simulink model "power_windgen_v2"  (R2021a)
settings: Solver=ode23tb  StartTime=0.0  StopTime=5  RelTol=1e-4  EnableMultiTasking=on
PostLoadFcn:
  | find_system (gcs, 'LookUnderMasks', 'all', 'FollowLinks', 'on');
InitFcn:
  | [xInitial,psbwindgen_char] = init_power_windgen;
undefined symbols (not defined in the file): DiscIntNeverNeededParam, psbwindgen_char
libraries: spsIdealSwitchLib x24, spsThreePhaseParallelRLCLoadLib x11, spsThreePhaseVIMeasurementLib x4, spsPower3phInstantaneousLib x4, spsThreePhaseBreakerLib x1, spsAsynchronousMachinepuUnitsLib x1, spsPLL3phLib x1, spsExcitationSystemLib x1, spsSynchronousMachinepuStandardLib x1, spspowerguiLib x1
Description:
  | The Model initialization function Callback automatically
  | 
  | loads the initial states vector xInitial and the wind turbine
  | 
  | characteristics. The initial conditions are stored in the
  | 
  | power_windgen.mat file.
settings Model: ExtModeAutoUpdateStatusClock=off  Creator=The MathWorks, Inc.  LastModifiedBy=enes_
settings SolverCC: AlgebraicLoopSolver=TrustRegion
settings DataIOCC: LoadInitialState=on  SaveFormat=StructureWithTime  SaveOutput=off  SaveTime=off  ReturnWorkspaceOutputs=off  SignalLoggingName=sigsOut
settings OptimizationCC: BlockReduction=off  BooleanDataType=off  ExpressionDepthLimit=2147483647  InitFltsAndDblsToZero=on  EfficientMapNaN2IntZero=off  LifeSpan=inf
settings DebuggingCC: UnderspecifiedInitializationDetection=Classic  MergeDetectMultiDrivingBlocksExec=none  CheckExecutionContextPreStartOutputMsg=on  SignalResolutionControl=TryResolveAllWithWarning  MultiTaskDSMMsg=warning  MultiTaskCondExecSysMsg=none  FcnCallInpInsideContextMsg=warning  AllowSymbolicDim=off  StateNameClashWarn=warning  SFUnexpectedBacktrackingDiag=warning  SFNoUnconditionalDefaultTransitionDiag=warning  SFExecutionAtInitializationDiag=none  SFMachineParentedDataDiag=warning  ArithmeticOperatorsInVariantConditions=warning
settings HardwareCC: ProdBitPerPointer=32  ProdBitPerSizeT=32  ProdBitPerPtrDiffT=32  ProdLargestAtomicFloat=None  ProdIntDivRoundTo=Undefined  ProdEndianess=Unspecified  ProdWordSize=32  ProdHWDeviceType=Specified  TargetUnknown=on
settings ModelReferenceCC: PropagateSignalLabelsOutOfModel=off
settings SFSimCC: SimUseLocalCustomCode=off  CustomCodeUndefinedFunction=UseInterfaceOnly
settings RTWCC: RTWUseLocalCustomCode=off
settings CodeAppCC: StateflowObjectComments=on
settings GRTTargetCC: TargetLangStandard=C89/C90 (ANSI)  CombineOutputUpdateFcns=off  GRTInterface=on
settings ConfigComp: CovMetricSettings=dw  CovSaveCumulativeToWorkspaceVar=on  CovSaveSingleToWorkspaceVar=on  CovExternalEMLEnable=off  CovSFcnEnable=off
settings SimscapeCC: SimscapeNormalizeSystem=off

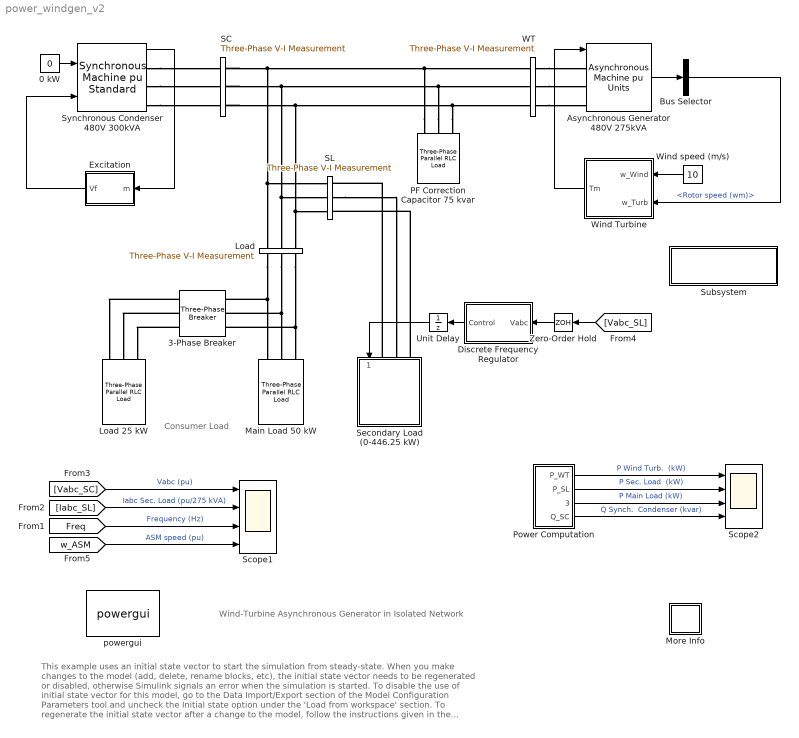
== system power_windgen_v2 ==
  note: This example uses an initial state vector to start the simulation from steady-state. When you make changes to the model (add, delete, rename blocks, etc),
      | the initial state vector needs to be regenerated or disabled, otherwise Simulink signals an error when the simulation is started.
      | To disable the use of initial state vector for this model, go to the Data Import/Export section of the Model Configuration Parameters tool and uncheck the
      | Initial state option under the 'Load from workspace' section.
      | To regenerate the initial state vector after a change to the model, follow the instructions given in the initialization file for this model.
      | Type open('init_power_windgen') at the matlab prompt to view this file.
  note: Wind-Turbine Asynchronous Generator in Isolated Network
  note: Consumer Load
  0 kW : Constant  Value=0
  3-Phase Breaker : spsThreePhaseBreakerLib/Three-Phase Breaker  InitialState=open  SwitchA=on  SwitchB=on  SwitchC=on  SwitchTimes=[0.2]  External=off  BreakerResistance=0.001  SnubberResistance=1e6  SnubberCapacitance=inf  Measurements=None
      settings: AttributesFormatString=\n
  Asynchronous Generator 480V 275kVA : spsAsynchronousMachinepuUnitsLib/Asynchronous Machine pu Units  RotorType=Squirrel-cage  PresetModel=No  MechanicalLoad=Torque Tm  ShowDetailedParameters=on  ReferenceFrame=Rotor  Units=pu  MeasurementBus=off  NominalParameters=[ 275e3, 480, 60 ]  VoltageRatio=1  Stator=[ 0.016,0.06]  Rotor=[ 0.015,0.06]  Cage1=[0.01909 0.0397]  Cage2=[0.01909 0.0397]  Lm=3.5  Mechanical=[ 2,0,2 ]  PolePairs=2  InitialConditions=[-8.89496e-048 0 0.280896 0.280896 0.280896 -89.7425 150.258 30.2575]  SimulateSaturation=off  Saturation=[ 0 0 ; 0 0 ]  LoadFlowParameters=0  TsPowergui=0  TsBlock=-1  IterativeModel=Trapezoidal non iterative  IterativeDiscreteModel=Trapezoidal non iterative  Pmec=0
      settings: AttributesFormatString=\n  SourceProductBaseCode=PS
  Bus Selector : BusSelector  OutputSignals=Mechanical.Rotor speed (wm)
  Discrete Frequency Regulator : Subsystem  mask(Discrete Frequency Regulator){Freq_ref=60, gains_regulator=[255 30], Vpp_nom=480, Ts=200e-6}
      mask prompts: Freq_ref "Reference frequency (Hz):"; gains_regulator "Regulator gains  [Kp Kd]:"; Vpp_nom "Phase to phase voltage (Vrms):"; Ts "Sample time (s):"
      mask help:
      | Input : phase to ground voltages
      |
      | Output : 24 logical signals for the control of the dump load
      mask init:
      | Vbase=Vpp_nom/sqrt(3);
      | Kp=gains_regulator(1);
      | Kd=gains_regulator(2);
  Excitation : Subsystem
  Load : spsThreePhaseVIMeasurementLib/Three-Phase V-I Measurement  VoltageMeasurement=phase-to-ground  SetLabelV=on  LabelV=Vabc_Load  Vpu=on  VpuLL=off  CurrentMeasurement=yes  SetLabelI=on  LabelI=Iabc_Load  Ipu=on  Pbase=275e3  Vbase=480  OutputType=Magnitude  PhasorSimulation=off  PSBequivalent=0
  Load 25 kW : spsThreePhaseParallelRLCLoadLib/Three-Phase Parallel RLC Load  LConnTagsString=A|B|C  Configuration=Y (grounded)  NominalVoltage=480  Vabc=[1e3 1e3 1e3]  Vabcp=[1e3 1e3 1e3]  NominalFrequency=60  UnbalancedPower=off  ActivePower=25e3  InductivePower=0  CapacitivePower=0  Pabc=[10e3 9e3 11e3]  QLabc=[100 90 110]  QCabc=[100 90 110]  Pabcp=[10e3 9e3 11e3]  QLabcp=[100 90 110]  QCabcp=[100 90 110]  Measurements=None  LoadType=constant Z
  Main Load 50 kW : spsThreePhaseParallelRLCLoadLib/Three-Phase Parallel RLC Load  LConnTagsString=A|B|C  Configuration=Y (grounded)  NominalVoltage=480  Vabc=[1e3 1e3 1e3]  Vabcp=[1e3 1e3 1e3]  NominalFrequency=60  UnbalancedPower=off  ActivePower=50e3  InductivePower=0  CapacitivePower=0  Pabc=[10e3 9e3 11e3]  QLabc=[100 90 110]  QCabc=[100 90 110]  Pabcp=[10e3 9e3 11e3]  QLabcp=[100 90 110]  QCabcp=[100 90 110]  Measurements=None  LoadType=constant Z
  More Info : Subsystem
      settings: OpenFcn=showdemo(bdroot(gcb))
      mask Display: disp('?')
  PF Correction Capacitor 75 kvar : spsThreePhaseParallelRLCLoadLib/Three-Phase Parallel RLC Load  LConnTagsString=A|B|C  Configuration=Delta  NominalVoltage=480  Vabc=[1e3 1e3 1e3]  Vabcp=[1e3 1e3 1e3]  NominalFrequency=60  UnbalancedPower=off  ActivePower=0  InductivePower=0  CapacitivePower=75e3  Pabc=[10e3 9e3 11e3]  QLabc=[100 90 110]  QCabc=[100 90 110]  Pabcp=[10e3 9e3 11e3]  QLabcp=[100 90 110]  QCabcp=[100 90 110]  Measurements=None  LoadType=constant Z
  Power Computation : Subsystem
  SC : spsThreePhaseVIMeasurementLib/Three-Phase V-I Measurement  VoltageMeasurement=phase-to-ground  SetLabelV=on  LabelV=Vabc_SC  Vpu=on  VpuLL=off  CurrentMeasurement=yes  SetLabelI=on  LabelI=Iabc_SC  Ipu=on  Pbase=300e3  Vbase=480  OutputType=Magnitude  PhasorSimulation=off  PSBequivalent=0
  SL : spsThreePhaseVIMeasurementLib/Three-Phase V-I Measurement  VoltageMeasurement=phase-to-ground  SetLabelV=on  LabelV=Vabc_SL  Vpu=on  VpuLL=off  CurrentMeasurement=yes  SetLabelI=on  LabelI=Iabc_SL  Ipu=on  Pbase=275e3  Vbase=480  OutputType=Magnitude  PhasorSimulation=off  PSBequivalent=0
  Scope1 : Scope  NumInputPorts=4
  Scope2 : Scope  NumInputPorts=4
  Secondary Load (0-446.25 kW) : Subsystem  mask(8-step Variable Load){Vphase_phase_lissage=480, Freq=60, P_lissage_min=1.75e3, Pin_3phase=50e3}
      mask prompts: Vphase_phase_lissage "Nominal L-L voltage (Vrms):"; Freq "Nominal frequency (Hz):"; P_lissage_min "Power per step Pstep (W):"; Pin_3phase "Initial power  (W) :"
      mask help:
      | This block implements a variable, three-phase resistive load. The load variation uses an eight-bit binary progression so that the load power can be varied by steps from 0 to 255*Pstep.
      |
      | The eight three-phase resistors are connected in series with ideal switches simulating forced-commutated power electronic switches.
      |
      | The Pulses input is a vector containing the eight bits (0/1) controlling the eight three-phase switches. First value is the less significant bit.
      mask init:
      | Ron_switch=1e-6;
      | Rs_snubber=inf;
      | Cs_snubber=0;
      | n_niveaux=8;
      | Pmax=((2^n_niveaux)-1)*P_lissage_min;
      | Pin_normalise=min([(Pin_3phase/Pmax)*((2^n_niveaux)-1) ((2^n_niveaux)-1)]);
      | discret1=pow2(0:-1:-(n_niveaux-1))*Pin_normalise;
      | discret2=floor(discret1);
      | Status=rem(discret2,2);
  Subsystem : Subsystem
      settings: OpenFcn=open('psbwindgen_turb.fig')
      mask Display: disp('Double click to display\nTurbine characteristics')
  Synchronous Condenser 480V 300kVA : spsSynchronousMachinepuStandardLib/Synchronous Machine pu Standard  PresetModel=No  MechanicalLoad=Mechanical power Pm  ShowDetailedParameters=on  RotorType=Salient-pole  Units=per unit standard parameters  MeasurementBus=off  NominalParameters=[ 300e3 480 60 ]  Reactances1=[ 3.23, 0.21, 0.15, 2.79, 1.03, 0.37, 0.09 ]  Reactances2=[2.24 0.17 0.12 1.02 0.13 0.08]  dAxisTimeConstants=Open-circuit  qAxisTimeConstants=Open-circuit  TimeConstants1="[ 4.4849  0.0681  0.1  ]"  TimeConstants2=[ 1.7, 0.008, 0.213, 0.004 ]  TimeConstants3="[  1.7 0.008 0.051266  ]"  TimeConstants4=[ 8.0, 0.03, 0.3371, 0.0295 ]  TimeConstants5="[ 0.08  0.019  0.004 ]"  TimeConstants6=[ 1.3201, 0.023, 1.0, 0.07 ]  TimeConstants7="[  0.08  0.019 0.051266  ]"  TimeConstants8=[ 1.3201, 0.0231, 0.3371, 0.0295 ]  StatorResistance=0.017  Mechanical=[ 1, 0, 2 ]  PolePairs=2  InitialConditions=[0 -89.2146 0.827 0.827 0.827 -86.4 153.6 33.6 2.71455]  SetSaturation=off  Saturation=[0.6404,0.7127,0.8441,0.9214,0.9956,1.082,1.19,1.316,1.457;0.7,0.7698,0.8872,0.9466,0.9969,1.046,1.1,1.151,1.201]  LoadFlowParameters=[2 0 0 0 0]  TsPowergui=0  TsBlock=-1  IterativeModel=Trapezoidal non iterative  IterativeDiscreteModel=Trapezoidal non iterative  BusType=PV  Pref=0  Qref=0  Qmin=-inf  Qmax=inf  PLF=0  QLF=0
      settings: SourceProductBaseCode=PS
  Unit Delay : UnitDelay  SampleTime=200e-6  HasFrameUpgradeWarning=on
  WT : spsThreePhaseVIMeasurementLib/Three-Phase V-I Measurement  VoltageMeasurement=phase-to-ground  SetLabelV=on  LabelV=Vabc_WT  Vpu=on  VpuLL=off  CurrentMeasurement=yes  SetLabelI=on  LabelI=Iabc_WT  Ipu=on  Pbase=275e3  Vbase=480  OutputType=Magnitude  PhasorSimulation=off  PSBequivalent=0
  Wind Turbine : Subsystem
  Wind speed (m/s) : Constant  Value=10
  Zero-Order Hold : ZeroOrderHold  SampleTime=200e-6
  powergui : spspowerguiLib/powergui  SimulationMode=Continuous  SampleTime=0  frequency=60  Iterations=50  frequencyindice=60  Pbase=100e6  ErrMax=1e-4  UnitsV=kV  UnitsW=MW  buscounter=0  FunctionMessages=off  echomessages=off  EnableUseOfTLC=off  CurrentSourceSwitches=on  DisableSnubberDevices=on  DisableRonSwitches=off  DisableVfSwitches=off  DisplayEquations=off  AutomaticDiscreteSolvers=off  SolverType=Tustin  Interpol=off  ExternalGateDelay=off  methode=off  Ts=0  x0status=blocks  SPID=off  SwTol=0  HookPort=off  NonlinearTolerance=1e-4  nMaxIteration=100  ContinueOnMaxIteration=off  RestoreLinks=warning  ResistiveCurrentMeasurement=off  Frange=[0:2:500]  Ylog=off  Xlog=on  ShowGrid=off  save=off  variable=ZData  structure=0  ZoomFFT=on  StartTime=0.0  cycles=1  DisplayStyle=1  fundamental=60  FreqAxis=off  MaxFrequency=1000  frequencyindicesteady=1  RmsSteady=1  display=off
  wires:
  [Freq] -> Scope1/3  "Frequency (Hz)"
  [Vabc_SC] -> Scope1/1  "Vabc (pu)"
  [Iabc_SL] -> Scope1/2  "Iabc Sec. Load (pu/275 kVA)"
  Wind speed (m/s)/1 -> Wind Turbine/1(w_Wind)
  [Vabc_SL] -> Zero-Order Hold/1
  Power Computation/1(P_WT) -> Scope2/1  "P Wind Turb.  (kW)"
  Power Computation/2(P_SL) -> Scope2/2  "P Sec. Load  (kW)"
  Power Computation/3(P_Load) -> Scope2/3  "P Main Load (kW)"
  Power Computation/4(Q_SC) -> Scope2/4  "Q Synch.  Condenser (kvar)"
  Discrete Frequency Regulator/1(Control) -> Unit Delay/1
  [w_ASM] -> Scope1/4  "ASM speed (pu)"
  0 kW/1 -> Synchronous Condenser 480V 300kVA/1
  Synchronous Condenser 480V 300kVA/1 -> Excitation/1(m)
  Excitation/1(Vf) -> Synchronous Condenser 480V 300kVA/2
  Asynchronous Generator 480V 275kVA/1 -> Bus Selector/1
  Wind Turbine/1(Tm) -> Asynchronous Generator 480V 275kVA/1
  Bus Selector/1 -> Wind Turbine/2(w_Turb)  "<Rotor speed (wm)>"
  Unit Delay/1 -> Secondary Load (0-446.25 kW)/1(Control)
  Zero-Order Hold/1 -> Discrete Frequency Regulator/1(Vabc)
  connections:
  Load/RConn3 -- Main Load 50 kW/LConn3 -- 3-Phase Breaker/LConn3
  Load/RConn1 -- Main Load 50 kW/LConn1 -- 3-Phase Breaker/LConn1
  Load/RConn2 -- Main Load 50 kW/LConn2 -- 3-Phase Breaker/LConn2
  WT/RConn1 -- Asynchronous Generator 480V 275kVA/LConn1
  WT/RConn2 -- Asynchronous Generator 480V 275kVA/LConn2
  WT/RConn3 -- Asynchronous Generator 480V 275kVA/LConn3
  Synchronous Condenser 480V 300kVA/RConn1 -- SC/LConn1
  Synchronous Condenser 480V 300kVA/RConn2 -- SC/LConn2
  Synchronous Condenser 480V 300kVA/RConn3 -- SC/LConn3
  PF Correction Capacitor 75 kvar/LConn1 -- WT/LConn1 -- SC/RConn1 -- Load/LConn1 -- SL/LConn1
  PF Correction Capacitor 75 kvar/LConn2 -- WT/LConn2 -- SC/RConn2 -- Load/LConn2 -- SL/LConn2
  PF Correction Capacitor 75 kvar/LConn3 -- WT/LConn3 -- SC/RConn3 -- Load/LConn3 -- SL/LConn3
  3-Phase Breaker/RConn1 -- Load 25 kW/LConn1
  3-Phase Breaker/RConn2 -- Load 25 kW/LConn2
  3-Phase Breaker/RConn3 -- Load 25 kW/LConn3
  Secondary Load (0-446.25 kW)/LConn1 -- SL/RConn1
  SL/RConn2 -- Secondary Load (0-446.25 kW)/LConn2
  Secondary Load (0-446.25 kW)/LConn3 -- SL/RConn3

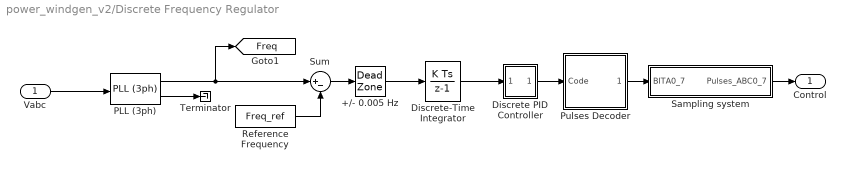
== system power_windgen_v2/Discrete Frequency Regulator ==
  Vabc : Inport
  +/- 0.005 Hz : DeadZone  LowerValue=-0.005  UpperValue=0.005  SaturateOnIntegerOverflow=on
  Discrete PID Controller : Subsystem  DialogController=POWERSYS.PowerSysDialog  mask(Discrete PID Controller){Kp=Kp, Ki=0, Kd=Kd, TcD=0.5e-3, Par_Limits=[255 0], Init=0, Ts=Ts}
      mask prompts: Kp "Proportional gain (Kp):"; Ki "Integral gain (Ki):"; Kd "Derivative gain (Kd):"; TcD "Time constant for derivative (s):"; Par_Limits "Output limits: [ Upper   Lower ]"; Init "Output initial value:"; Ts "Sample time:"
      mask help: This block implements a discrete PID controller.
      mask init:
      | UpperLimit=Par_Limits(1);
      | LowerLimit=Par_Limits(2);
      | power_initmask();
      mask Help: This block is part of a subset of blocks in the Extras library that does not have documentation associated with it, other than the block mask description.
      mask Display: disp('PID');
  Discrete-Time Integrator : DiscreteIntegrator  SampleTime=Ts  LimitOutput=on  UpperSaturationLimit=1  LowerSaturationLimit=0  ICPrevOutput=DiscIntNeverNeededParam  ICPrevScaledInput=DiscIntNeverNeededParam
  PLL (3ph) : spsPLL3phLib/PLL (3ph)  Fmin=45  Par_Init=[0 Freq_ref]  ParK=[60 1400]  TcD=2e-4  MaxRateChangeFreq=12  FilterCutOffFreq=25  Ts=Ts  AGC=on
  Pulses Decoder : Subsystem  mask(Pulses Decoder){n=8}
      mask prompts: n "Number of bits to decode:"
      mask help:
      | Decode the scalar input 'Code' into a vector output 'Pulses' based on  the specified number of bits to decode.
      | (Element 1 of vector output = least significant bit)
  Reference Frequency : Constant  Value=Freq_ref
  Sampling system : Subsystem
  Sum : Sum  Inputs=|+-  InputSameDT=on  SaturateOnIntegerOverflow=on  OutDataTypeStr=Inherit: Same as first input
  Terminator : Terminator
  Control : Outport  VectorParamsAs1DForOutWhenUnconnected=off
  tag scope: Freq=global
  wires:
  Vabc/1 -> PLL (3ph)/1
  PLL (3ph)/2 -> Terminator/1
  Sampling system/1(Pulses_ABC0_7) -> Control/1
  Discrete-Time Integrator/1 -> Discrete PID Controller/1(Error)
  Reference Frequency/1 -> Sum/2
  Discrete PID Controller/1(Out) -> Pulses Decoder/1(Code)
  Sum/1 -> +/- 0.005 Hz/1
  Pulses Decoder/1(Pulses) -> Sampling system/1(BITA0_7)
  +/- 0.005 Hz/1 -> Discrete-Time Integrator/1
  PLL (3ph)/1 -> Sum/1, [Freq]

== system power_windgen_v2/Excitation ==
  m : Inport
  Bus Selector1 : BusSelector  OutputSignals="dq0 components.Stator voltage  vd (pu),dq0 components.Stator voltage  vq (pu)"
  Constant3 : Constant
  Excitation System : spsExcitationSystemLib/Excitation System  tr=20e-3  reg=[ 300, 0.001 ]  exc=[ 1, 0 ]  tgr=[ 0, 0 ]  damp=[ 0.001, 0.1 ]  sat=[ 0, 0 ]  lim=[ -11.5, 11.5, 0 ]  v0=[1,2.71455]
      settings: SourceProductBaseCode=PS
  Ground : Ground
  Vf : Outport  VectorParamsAs1DForOutWhenUnconnected=off
  wires:
  Constant3/1 -> Excitation System/1
  Ground/1 -> Excitation System/4
  m/1 -> Bus Selector1/1
  Excitation System/1 -> Vf/1
  Bus Selector1/1 -> Excitation System/2  "<Stator voltage  vd (pu)>"
  Bus Selector1/2 -> Excitation System/3  "<Stator voltage  vq (pu)>"

== system power_windgen_v2/More Info ==

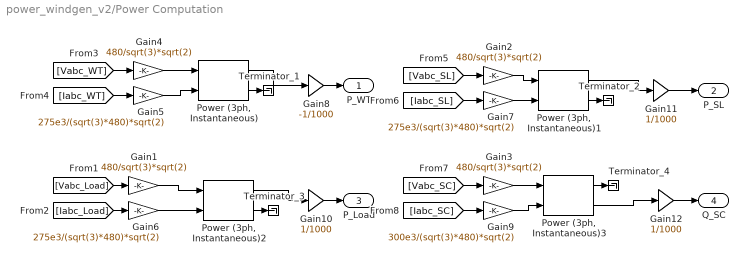
== system power_windgen_v2/Power Computation ==
  Gain{1..4} (4 alike) : Gain  Gain=480/sqrt(3)*sqrt(2)  SaturateOnIntegerOverflow=on  OutDataTypeStr=Inherit: Same as input  ParamDataTypeStr=Inherit: Same as input
  Gain10 : Gain  Gain=1/1000  SaturateOnIntegerOverflow=on  OutDataTypeStr=Inherit: Same as input  ParamDataTypeStr=Inherit: Same as input
  Gain11 : Gain  Gain=1/1000  SaturateOnIntegerOverflow=on  OutDataTypeStr=Inherit: Same as input  ParamDataTypeStr=Inherit: Same as input
  Gain12 : Gain  Gain=1/1000  SaturateOnIntegerOverflow=on  OutDataTypeStr=Inherit: Same as input  ParamDataTypeStr=Inherit: Same as input
  Gain5 : Gain  Gain=275e3/(sqrt(3)*480)*sqrt(2)  SaturateOnIntegerOverflow=on  OutDataTypeStr=Inherit: Same as input  ParamDataTypeStr=Inherit: Same as input
  Gain6 : Gain  Gain=275e3/(sqrt(3)*480)*sqrt(2)  SaturateOnIntegerOverflow=on  OutDataTypeStr=Inherit: Same as input  ParamDataTypeStr=Inherit: Same as input
  Gain7 : Gain  Gain=275e3/(sqrt(3)*480)*sqrt(2)  SaturateOnIntegerOverflow=on  OutDataTypeStr=Inherit: Same as input  ParamDataTypeStr=Inherit: Same as input
  Gain8 : Gain  Gain=-1/1000  SaturateOnIntegerOverflow=on  OutDataTypeStr=Inherit: Same as input  ParamDataTypeStr=Inherit: Same as input
  Gain9 : Gain  Gain=300e3/(sqrt(3)*480)*sqrt(2)  SaturateOnIntegerOverflow=on  OutDataTypeStr=Inherit: Same as input  ParamDataTypeStr=Inherit: Same as input
  Power (3ph, Instantaneous){,1..3} (4 alike) : spsPower3phInstantaneousLib/Power (3ph, Instantaneous)
  Terminator_{1..4} (4 alike) : Terminator
  P_WT : Outport  VectorParamsAs1DForOutWhenUnconnected=off
  P_SL : Outport  Port=2  VectorParamsAs1DForOutWhenUnconnected=off
  P_Load : Outport  Port=3  VectorParamsAs1DForOutWhenUnconnected=off
  Q_SC : Outport  Port=4  VectorParamsAs1DForOutWhenUnconnected=off
  wires:
  "Power (3ph, Instantaneous)1"/1 -> Gain11/1
  [Vabc_WT] -> Gain4/1
  [Iabc_WT] -> Gain5/1
  Gain4/1 -> "Power (3ph, Instantaneous)"/1
  Gain5/1 -> "Power (3ph, Instantaneous)"/2
  [Vabc_Load] -> Gain1/1
  [Iabc_Load] -> Gain6/1
  Gain1/1 -> "Power (3ph, Instantaneous)2"/1
  Gain6/1 -> "Power (3ph, Instantaneous)2"/2
  [Vabc_SL] -> Gain2/1
  [Iabc_SL] -> Gain7/1
  Gain2/1 -> "Power (3ph, Instantaneous)1"/1
  Gain7/1 -> "Power (3ph, Instantaneous)1"/2
  "Power (3ph, Instantaneous)2"/1 -> Gain10/1
  "Power (3ph, Instantaneous)"/1 -> Gain8/1
  Gain8/1 -> P_WT/1
  "Power (3ph, Instantaneous)3"/2 -> Gain12/1
  [Vabc_SC] -> Gain3/1
  [Iabc_SC] -> Gain9/1
  Gain3/1 -> "Power (3ph, Instantaneous)3"/1
  Gain9/1 -> "Power (3ph, Instantaneous)3"/2
  Gain10/1 -> P_Load/1
  Gain11/1 -> P_SL/1
  Gain12/1 -> Q_SC/1
  "Power (3ph, Instantaneous)"/2 -> Terminator_1/1
  "Power (3ph, Instantaneous)1"/2 -> Terminator_2/1
  "Power (3ph, Instantaneous)2"/2 -> Terminator_3/1
  "Power (3ph, Instantaneous)3"/1 -> Terminator_4/1

== system power_windgen_v2/Secondary Load (0-446.25 kW) ==
  Control : Inport
  Demux : Demux  Outputs=8
      settings: DisplayOption=none
  Resistive Loads : Subsystem
  Switches : Subsystem
  A : PMIOPort  Side=Left
  B : PMIOPort  Port=2  Side=Left
  C : PMIOPort  Port=3  Side=Left
  wires:
  Control/1 -> Demux/1
  Demux/8 -> Switches/8(P_ABC7)
  Demux/7 -> Switches/7(P_ABC6)
  Demux/6 -> Switches/6(P_ABC5)
  Demux/5 -> Switches/5(P_ABC4)
  Demux/4 -> Switches/4(P_ABC3)
  Demux/3 -> Switches/3(P_ABC2)
  Demux/2 -> Switches/2(P_ABC1)
  Demux/1 -> Switches/1(P_ABC0)
  connections:
  Switches/RConn1 -- Resistive Loads/LConn1
  Switches/RConn2 -- Resistive Loads/LConn2
  Switches/RConn3 -- Resistive Loads/LConn3
  Switches/RConn4 -- Resistive Loads/LConn4
  Switches/RConn5 -- Resistive Loads/LConn5
  Switches/RConn6 -- Resistive Loads/LConn6
  Switches/RConn7 -- Resistive Loads/LConn7
  Switches/RConn8 -- Resistive Loads/LConn8
  Switches/RConn9 -- Resistive Loads/LConn9
  Switches/RConn10 -- Resistive Loads/LConn10
  Switches/RConn11 -- Resistive Loads/LConn11
  Switches/RConn12 -- Resistive Loads/LConn12
  Switches/RConn13 -- Resistive Loads/LConn13
  Switches/RConn14 -- Resistive Loads/LConn14
  Switches/RConn15 -- Resistive Loads/LConn15
  Switches/RConn16 -- Resistive Loads/LConn16
  Switches/RConn17 -- Resistive Loads/LConn17
  Switches/RConn18 -- Resistive Loads/LConn18
  Switches/RConn19 -- Resistive Loads/LConn19
  Switches/RConn20 -- Resistive Loads/LConn20
  Switches/RConn21 -- Resistive Loads/LConn21
  Switches/RConn22 -- Resistive Loads/LConn22
  Switches/RConn23 -- Resistive Loads/LConn23
  Switches/RConn24 -- Resistive Loads/LConn24
  A/RConn1 -- Switches/LConn1
  B/RConn1 -- Switches/LConn2
  C/RConn1 -- Switches/LConn3

== system power_windgen_v2/Subsystem ==

== system power_windgen_v2/Wind Turbine ==
  w_Wind : Inport
  w_Turb : Inport  Port=2
  1800 rpm : Gain  Gain=1800  SaturateOnIntegerOverflow=on  OutDataTypeStr=Inherit: Same as input  ParamDataTypeStr=Inherit: Same as input
  Constant3 : Constant  Value=1e-6
  Gain : Gain  Gain=-1  SaturateOnIntegerOverflow=on  OutDataTypeStr=Inherit: Same as input  ParamDataTypeStr=Inherit: Same as input
  P(w_Wind,w_Turb) : Lookup_n-D  BreakpointsForDimension1=[0 5 6 7 8 9 10 11 12]  BreakpointsForDimension2=[0 571.55 685.8 800.15 914.4 1028.8 1143.1 1257.4 1371.7 1486 1600.3 1714.6 1828.9 1943.2 2057.5 2171.8 2286.1 2400.5 2514.7 2629.1 2743.3 2857.7 2971.9 3086.3 3200.5 3314.9 3429.2]  Table=psbwindgen_char  InternalRulePriority=Speed  RndMeth=Simplest  InputSameDT=on
      settings: InputPortMap=u0,u1
  Product : Product  Inputs=*/  InputSameDT=on  SaturateOnIntegerOverflow=on  OutDataTypeStr=Inherit: Same as first input
  Switch : Switch  Threshold=1e-6  SaturateOnIntegerOverflow=on  InputSameDT=on
  Tm : Outport  VectorParamsAs1DForOutWhenUnconnected=off
  tag scope: w_ASM=global
  wires:
  w_Turb/1 -> 1800 rpm/1, Switch/1, Switch/2, [w_ASM]
  Constant3/1 -> Switch/3
  w_Wind/1 -> P(w_Wind,w_Turb)/1
  P(w_Wind,w_Turb)/1 -> Product/1
  Switch/1 -> Product/2
  Product/1 -> Gain/1
  Gain/1 -> Tm/1
  1800 rpm/1 -> P(w_Wind,w_Turb)/2

== system power_windgen_v2/Discrete Frequency Regulator/Discrete PID Controller ==
  note: Pierre Giroux, Gilbert Sybille
      | Power System Simulation Laboratory
      | IREQ, Hydro-Quebc
  note: Discrete PID Controller
  Error : Inport  SampleTime=Ts
  "Derivative " : DiscreteTransferFcn  Numerator=[2 -2]  Denominator=[Ts+2*TcD Ts-2*TcD]  SampleTime=Ts
  Discrete-Time Integrator : DiscreteIntegrator  InitialCondition=Init  SampleTime=Ts  LimitOutput=on  UpperSaturationLimit=UpperLimit  LowerSaturationLimit=LowerLimit  ICPrevOutput=DiscIntNeverNeededParam  ICPrevScaledInput=DiscIntNeverNeededParam
  Kp4 : Gain  Gain=Kp  SaturateOnIntegerOverflow=on  SampleTime=Ts  OutDataTypeStr=Inherit: Same as input  ParamDataTypeStr=Inherit: Same as input
  Kp5 : Gain  Gain=Ki  SaturateOnIntegerOverflow=on  SampleTime=Ts  OutDataTypeStr=Inherit: Same as input  ParamDataTypeStr=Inherit: Same as input
  Kp6 : Gain  Gain=Kd  SaturateOnIntegerOverflow=on  SampleTime=Ts  OutDataTypeStr=Inherit: Same as input  ParamDataTypeStr=Inherit: Same as input
  Saturation2 : Saturate  UpperLimit=UpperLimit  LowerLimit=LowerLimit  SampleTime=Ts
  Sum6 : Sum  Inputs=+++  InputSameDT=on  SaturateOnIntegerOverflow=on  SampleTime=Ts  OutDataTypeStr=Inherit: Same as first input
  Zero-Order Hold : ZeroOrderHold  SampleTime=Ts
  Out : Outport  SampleTime=Ts  InitialOutput=0  VectorParamsAs1DForOutWhenUnconnected=off
  wires:
  Saturation2/1 -> Out/1
  Error/1 -> Kp4/1, Kp5/1, Kp6/1
  Sum6/1 -> Saturation2/1
  Kp5/1 -> Discrete-Time Integrator/1
  Kp6/1 -> "Derivative "/1
  Kp4/1 -> Zero-Order Hold/1
  Discrete-Time Integrator/1 -> Sum6/2
  "Derivative "/1 -> Sum6/3
  Zero-Order Hold/1 -> Sum6/1

== system power_windgen_v2/Discrete Frequency Regulator/Pulses Decoder ==
  Code : Inport
  Constant : Constant  Value=pow2(0:-1:-(n-1))
  Constant6 : Constant  Value=2
  Math Function : Math  Operator=rem  SignedPower=on  SaturateOnIntegerOverflow=on
  Product : Product  InputSameDT=on  SaturateOnIntegerOverflow=on  OutDataTypeStr=Inherit: Same as first input
  Rounding Function : Rounding
  Pulses : Outport  VectorParamsAs1DForOutWhenUnconnected=off
  wires:
  Math Function/1 -> Pulses/1
  Rounding Function/1 -> Math Function/1
  Constant6/1 -> Math Function/2
  Product/1 -> Rounding Function/1
  Code/1 -> Product/1
  Constant/1 -> Product/2

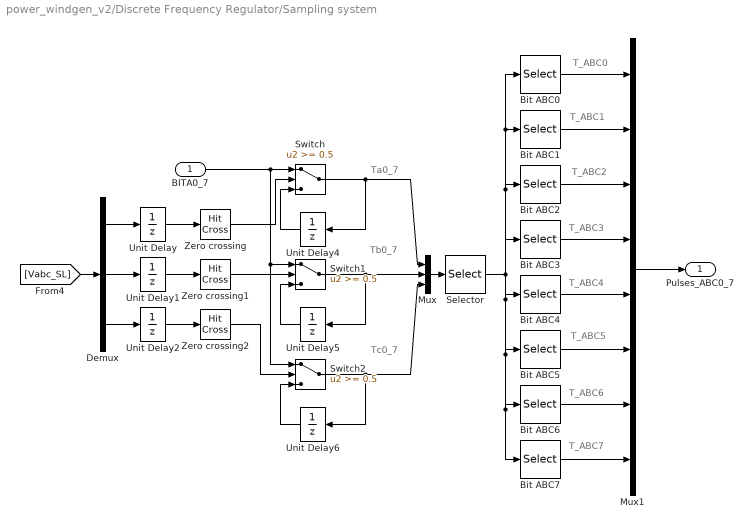
== system power_windgen_v2/Discrete Frequency Regulator/Sampling system ==
  note: T_ABC7
  note: T_ABC6
  note: T_ABC5
  note: T_ABC4
  note: T_ABC3
  note: T_ABC2
  note: T_ABC1
  note: T_ABC0
  note: Tc0_7
  note: Tb0_7
  note: Ta0_7
  BITA0_7 : Inport
  " Bit ABC4" : Selector  InputPortWidth=24  IndexOptions=Index vector (dialog)  Indices=[13 14 15]  OutputSizes=1
  Bit ABC0 : Selector  InputPortWidth=24  IndexOptions=Index vector (dialog)  Indices=[1 2 3]  OutputSizes=1
  Bit ABC1 : Selector  InputPortWidth=24  IndexOptions=Index vector (dialog)  Indices=[4 5 6]  OutputSizes=1
  Bit ABC2 : Selector  InputPortWidth=24  IndexOptions=Index vector (dialog)  Indices=[7 8 9]  OutputSizes=1
  Bit ABC3 : Selector  InputPortWidth=24  IndexOptions=Index vector (dialog)  Indices=[10 11 12]  OutputSizes=1
  Bit ABC5 : Selector  InputPortWidth=24  IndexOptions=Index vector (dialog)  Indices=[16 17 18]  OutputSizes=1
  Bit ABC6 : Selector  InputPortWidth=24  IndexOptions=Index vector (dialog)  Indices=[19 20 21]  OutputSizes=1
  Bit ABC7 : Selector  InputPortWidth=24  IndexOptions=Index vector (dialog)  Indices=[22 23 24]  OutputSizes=1
  Demux : Demux  Outputs=3
      settings: DisplayOption=none
  Mux : Mux  Inputs=3
  Mux1 : Mux  Inputs=8
  Selector : Selector  InputPortWidth=24  IndexOptions=Index vector (dialog)  Indices=[1 9 17 2 10 18 3 11 19 4 12 20 5 13 21 6 14 22 7 15 23 8 16 24]  OutputSizes=1
  Switch : Switch  Threshold=0.5  SaturateOnIntegerOverflow=on  InputSameDT=on
  Switch1 : Switch  Threshold=0.5  SaturateOnIntegerOverflow=on  InputSameDT=on
  Switch2 : Switch  Threshold=0.5  SaturateOnIntegerOverflow=on  InputSameDT=on
  Unit Delay{,1..2,4..6} (6 alike) : UnitDelay  SampleTime=Ts  HasFrameUpgradeWarning=on
  Zero crossing : HitCross
  Zero crossing1 : HitCross
  Zero crossing2 : HitCross
  Pulses_ABC0_7 : Outport  VectorParamsAs1DForOutWhenUnconnected=off
  wires:
  BITA0_7/1 -> Switch2/1, Switch1/1, Switch/1
  Demux/3 -> Unit Delay2/1
  Demux/2 -> Unit Delay1/1
  Demux/1 -> Unit Delay/1
  Mux1/1 -> Pulses_ABC0_7/1
  Bit ABC7/1 -> Mux1/8
  Bit ABC6/1 -> Mux1/7
  Bit ABC5/1 -> Mux1/6
  " Bit ABC4"/1 -> Mux1/5
  Bit ABC3/1 -> Mux1/4
  Bit ABC2/1 -> Mux1/3
  Bit ABC1/1 -> Mux1/2
  Bit ABC0/1 -> Mux1/1
  Selector/1 -> Bit ABC7/1, Bit ABC6/1, Bit ABC5/1, " Bit ABC4"/1, Bit ABC3/1, Bit ABC2/1, Bit ABC0/1, Bit ABC1/1
  Mux/1 -> Selector/1
  Unit Delay6/1 -> Switch2/3
  Switch2/1 -> Mux/3, Unit Delay6/1
  Unit Delay5/1 -> Switch1/3
  Switch1/1 -> Mux/2, Unit Delay5/1
  Unit Delay4/1 -> Switch/3
  Switch/1 -> Mux/1, Unit Delay4/1
  Unit Delay/1 -> Zero crossing/1
  Unit Delay2/1 -> Zero crossing2/1
  Zero crossing/1 -> Switch/2
  Zero crossing1/1 -> Switch1/2
  Zero crossing2/1 -> Switch2/2
  [Vabc_SL] -> Demux/1
  Unit Delay1/1 -> Zero crossing1/1

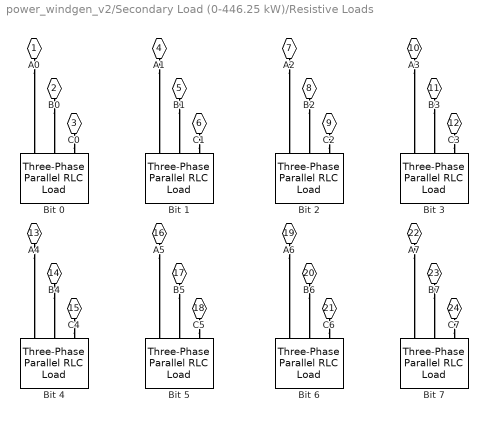
== system power_windgen_v2/Secondary Load (0-446.25 kW)/Resistive Loads ==
  Bit 0 : spsThreePhaseParallelRLCLoadLib/Three-Phase Parallel RLC Load  LConnTagsString=A|B|C  Configuration=Y (grounded)  NominalVoltage=Vphase_phase_lissage  Vabc=[1e3 1e3 1e3]  Vabcp=[1e3 1e3 1e3]  NominalFrequency=Freq  UnbalancedPower=off  ActivePower=P_lissage_min  InductivePower=0  CapacitivePower=0  Pabc=[10e3 9e3 11e3]  QLabc=[100 90 110]  QCabc=[100 90 110]  Pabcp=[10e3 9e3 11e3]  QLabcp=[100 90 110]  QCabcp=[100 90 110]  Measurements=None  LoadType=constant Z
  Bit 1 : spsThreePhaseParallelRLCLoadLib/Three-Phase Parallel RLC Load  LConnTagsString=A|B|C  Configuration=Y (grounded)  NominalVoltage=Vphase_phase_lissage  Vabc=[1e3 1e3 1e3]  Vabcp=[1e3 1e3 1e3]  NominalFrequency=Freq  UnbalancedPower=off  ActivePower=2*P_lissage_min  InductivePower=0  CapacitivePower=0  Pabc=[10e3 9e3 11e3]  QLabc=[100 90 110]  QCabc=[100 90 110]  Pabcp=[10e3 9e3 11e3]  QLabcp=[100 90 110]  QCabcp=[100 90 110]  Measurements=None  LoadType=constant Z
  Bit 2 : spsThreePhaseParallelRLCLoadLib/Three-Phase Parallel RLC Load  LConnTagsString=A|B|C  Configuration=Y (grounded)  NominalVoltage=Vphase_phase_lissage  Vabc=[1e3 1e3 1e3]  Vabcp=[1e3 1e3 1e3]  NominalFrequency=Freq  UnbalancedPower=off  ActivePower=2^2*P_lissage_min  InductivePower=0  CapacitivePower=0  Pabc=[10e3 9e3 11e3]  QLabc=[100 90 110]  QCabc=[100 90 110]  Pabcp=[10e3 9e3 11e3]  QLabcp=[100 90 110]  QCabcp=[100 90 110]  Measurements=None  LoadType=constant Z
  Bit 3 : spsThreePhaseParallelRLCLoadLib/Three-Phase Parallel RLC Load  LConnTagsString=A|B|C  Configuration=Y (grounded)  NominalVoltage=Vphase_phase_lissage  Vabc=[1e3 1e3 1e3]  Vabcp=[1e3 1e3 1e3]  NominalFrequency=Freq  UnbalancedPower=off  ActivePower=2^3*P_lissage_min  InductivePower=0  CapacitivePower=0  Pabc=[10e3 9e3 11e3]  QLabc=[100 90 110]  QCabc=[100 90 110]  Pabcp=[10e3 9e3 11e3]  QLabcp=[100 90 110]  QCabcp=[100 90 110]  Measurements=None  LoadType=constant Z
  Bit 4 : spsThreePhaseParallelRLCLoadLib/Three-Phase Parallel RLC Load  LConnTagsString=A|B|C  Configuration=Y (grounded)  NominalVoltage=Vphase_phase_lissage  Vabc=[1e3 1e3 1e3]  Vabcp=[1e3 1e3 1e3]  NominalFrequency=Freq  UnbalancedPower=off  ActivePower=2^4*P_lissage_min  InductivePower=0  CapacitivePower=0  Pabc=[10e3 9e3 11e3]  QLabc=[100 90 110]  QCabc=[100 90 110]  Pabcp=[10e3 9e3 11e3]  QLabcp=[100 90 110]  QCabcp=[100 90 110]  Measurements=None  LoadType=constant Z
  Bit 5 : spsThreePhaseParallelRLCLoadLib/Three-Phase Parallel RLC Load  LConnTagsString=A|B|C  Configuration=Y (grounded)  NominalVoltage=Vphase_phase_lissage  Vabc=[1e3 1e3 1e3]  Vabcp=[1e3 1e3 1e3]  NominalFrequency=Freq  UnbalancedPower=off  ActivePower=2^5*P_lissage_min  InductivePower=0  CapacitivePower=0  Pabc=[10e3 9e3 11e3]  QLabc=[100 90 110]  QCabc=[100 90 110]  Pabcp=[10e3 9e3 11e3]  QLabcp=[100 90 110]  QCabcp=[100 90 110]  Measurements=None  LoadType=constant Z
  Bit 6 : spsThreePhaseParallelRLCLoadLib/Three-Phase Parallel RLC Load  LConnTagsString=A|B|C  Configuration=Y (grounded)  NominalVoltage=Vphase_phase_lissage  Vabc=[1e3 1e3 1e3]  Vabcp=[1e3 1e3 1e3]  NominalFrequency=Freq  UnbalancedPower=off  ActivePower=2^6*P_lissage_min  InductivePower=0  CapacitivePower=0  Pabc=[10e3 9e3 11e3]  QLabc=[100 90 110]  QCabc=[100 90 110]  Pabcp=[10e3 9e3 11e3]  QLabcp=[100 90 110]  QCabcp=[100 90 110]  Measurements=None  LoadType=constant Z
  Bit 7 : spsThreePhaseParallelRLCLoadLib/Three-Phase Parallel RLC Load  LConnTagsString=A|B|C  Configuration=Y (grounded)  NominalVoltage=Vphase_phase_lissage  Vabc=[1e3 1e3 1e3]  Vabcp=[1e3 1e3 1e3]  NominalFrequency=Freq  UnbalancedPower=off  ActivePower=2^7*P_lissage_min  InductivePower=0  CapacitivePower=0  Pabc=[10e3 9e3 11e3]  QLabc=[100 90 110]  QCabc=[100 90 110]  Pabcp=[10e3 9e3 11e3]  QLabcp=[100 90 110]  QCabcp=[100 90 110]  Measurements=None  LoadType=constant Z
  A0 : PMIOPort  Side=Left
  B0 : PMIOPort  Port=2  Side=Left
  C0 : PMIOPort  Port=3  Side=Left
  A1 : PMIOPort  Port=4  Side=Left
  B1 : PMIOPort  Port=5  Side=Left
  C1 : PMIOPort  Port=6  Side=Left
  A2 : PMIOPort  Port=7  Side=Left
  B2 : PMIOPort  Port=8  Side=Left
  C2 : PMIOPort  Port=9  Side=Left
  A3 : PMIOPort  Port=10  Side=Left
  B3 : PMIOPort  Port=11  Side=Left
  C3 : PMIOPort  Port=12  Side=Left
  A4 : PMIOPort  Port=13  Side=Left
  B4 : PMIOPort  Port=14  Side=Left
  C4 : PMIOPort  Port=15  Side=Left
  A5 : PMIOPort  Port=16  Side=Left
  B5 : PMIOPort  Port=17  Side=Left
  C5 : PMIOPort  Port=18  Side=Left
  A6 : PMIOPort  Port=19  Side=Left
  B6 : PMIOPort  Port=20  Side=Left
  C6 : PMIOPort  Port=21  Side=Left
  A7 : PMIOPort  Port=22  Side=Left
  B7 : PMIOPort  Port=23  Side=Left
  C7 : PMIOPort  Port=24  Side=Left
  connections:
  C7/RConn1 -- Bit 7/LConn3
  B7/RConn1 -- Bit 7/LConn2
  A7/RConn1 -- Bit 7/LConn1
  C6/RConn1 -- Bit 6/LConn3
  B6/RConn1 -- Bit 6/LConn2
  A6/RConn1 -- Bit 6/LConn1
  C5/RConn1 -- Bit 5/LConn3
  B5/RConn1 -- Bit 5/LConn2
  A5/RConn1 -- Bit 5/LConn1
  C4/RConn1 -- Bit 4/LConn3
  B4/RConn1 -- Bit 4/LConn2
  A4/RConn1 -- Bit 4/LConn1
  C3/RConn1 -- Bit 3/LConn3
  B3/RConn1 -- Bit 3/LConn2
  A3/RConn1 -- Bit 3/LConn1
  C2/RConn1 -- Bit 2/LConn3
  B2/RConn1 -- Bit 2/LConn2
  A2/RConn1 -- Bit 2/LConn1
  C1/RConn1 -- Bit 1/LConn3
  B1/RConn1 -- Bit 1/LConn2
  A1/RConn1 -- Bit 1/LConn1
  C0/RConn1 -- Bit 0/LConn3
  B0/RConn1 -- Bit 0/LConn2
  A0/RConn1 -- Bit 0/LConn1

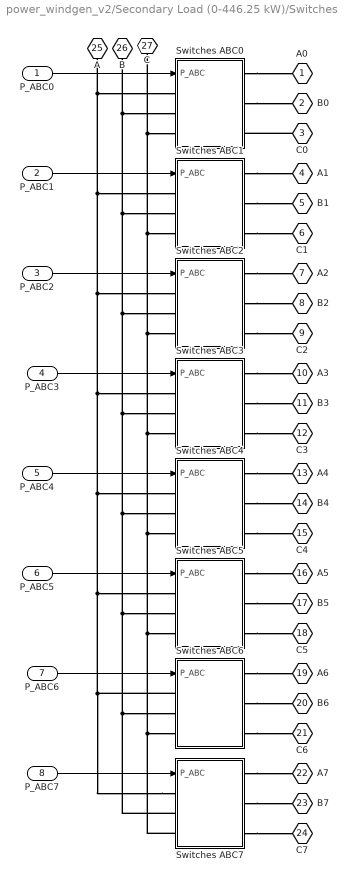
== system power_windgen_v2/Secondary Load (0-446.25 kW)/Switches ==
  P_ABC0 : Inport
  P_ABC1 : Inport  Port=2
  P_ABC2 : Inport  Port=3
  P_ABC3 : Inport  Port=4
  P_ABC4 : Inport  Port=5
  P_ABC5 : Inport  Port=6
  P_ABC6 : Inport  Port=7
  P_ABC7 : Inport  Port=8
  Switches ABC0 : Subsystem
  Switches ABC1 : Subsystem
  Switches ABC2 : Subsystem
  Switches ABC3 : Subsystem
  Switches ABC4 : Subsystem
  Switches ABC5 : Subsystem
  Switches ABC6 : Subsystem
  Switches ABC7 : Subsystem
  A0 : PMIOPort  Side=Right
  B0 : PMIOPort  Port=2  Side=Right
  C0 : PMIOPort  Port=3  Side=Right
  A1 : PMIOPort  Port=4  Side=Right
  B1 : PMIOPort  Port=5  Side=Right
  C1 : PMIOPort  Port=6  Side=Right
  A2 : PMIOPort  Port=7  Side=Right
  B2 : PMIOPort  Port=8  Side=Right
  C2 : PMIOPort  Port=9  Side=Right
  A3 : PMIOPort  Port=10  Side=Right
  B3 : PMIOPort  Port=11  Side=Right
  C3 : PMIOPort  Port=12  Side=Right
  A4 : PMIOPort  Port=13  Side=Right
  B4 : PMIOPort  Port=14  Side=Right
  C4 : PMIOPort  Port=15  Side=Right
  A5 : PMIOPort  Port=16  Side=Right
  B5 : PMIOPort  Port=17  Side=Right
  C5 : PMIOPort  Port=18  Side=Right
  A6 : PMIOPort  Port=19  Side=Right
  B6 : PMIOPort  Port=20  Side=Right
  C6 : PMIOPort  Port=21  Side=Right
  A7 : PMIOPort  Port=22  Side=Right
  B7 : PMIOPort  Port=23  Side=Right
  C7 : PMIOPort  Port=24  Side=Right
  A : PMIOPort  Port=25  Side=Left
  B : PMIOPort  Port=26  Side=Left
  C : PMIOPort  Port=27  Side=Left
  wires:
  P_ABC7/1 -> Switches ABC7/1(P_ABC)
  P_ABC6/1 -> Switches ABC6/1(P_ABC)
  P_ABC5/1 -> Switches ABC5/1(P_ABC)
  P_ABC4/1 -> Switches ABC4/1(P_ABC)
  P_ABC3/1 -> Switches ABC3/1(P_ABC)
  P_ABC2/1 -> Switches ABC2/1(P_ABC)
  P_ABC1/1 -> Switches ABC1/1(P_ABC)
  P_ABC0/1 -> Switches ABC0/1(P_ABC)
  connections:
  Switches ABC0/RConn1 -- A0/RConn1
  Switches ABC0/RConn2 -- B0/RConn1
  C0/RConn1 -- Switches ABC0/RConn3
  Switches ABC1/RConn1 -- A1/RConn1
  Switches ABC1/RConn2 -- B1/RConn1
  Switches ABC1/RConn3 -- C1/RConn1
  Switches ABC2/RConn1 -- A2/RConn1
  Switches ABC2/RConn2 -- B2/RConn1
  Switches ABC2/RConn3 -- C2/RConn1
  Switches ABC3/RConn1 -- A3/RConn1
  Switches ABC3/RConn2 -- B3/RConn1
  Switches ABC3/RConn3 -- C3/RConn1
  Switches ABC4/RConn1 -- A4/RConn1
  Switches ABC4/RConn2 -- B4/RConn1
  Switches ABC4/RConn3 -- C4/RConn1
  Switches ABC5/RConn1 -- A5/RConn1
  Switches ABC5/RConn2 -- B5/RConn1
  Switches ABC5/RConn3 -- C5/RConn1
  Switches ABC6/RConn1 -- A6/RConn1
  Switches ABC6/RConn2 -- B6/RConn1
  Switches ABC6/RConn3 -- C6/RConn1
  Switches ABC7/RConn3 -- C7/RConn1
  Switches ABC7/RConn2 -- B7/RConn1
  Switches ABC7/RConn1 -- A7/RConn1
  Switches ABC7/LConn2 -- Switches ABC0/LConn2 -- B/RConn1 -- Switches ABC1/LConn2 -- Switches ABC2/LConn2 -- Switches ABC3/LConn2 -- Switches ABC4/LConn2 -- Switches ABC5/LConn2 -- Switches ABC6/LConn2
  Switches ABC7/LConn3 -- Switches ABC0/LConn3 -- C/RConn1 -- Switches ABC1/LConn3 -- Switches ABC2/LConn3 -- Switches ABC3/LConn3 -- Switches ABC4/LConn3 -- Switches ABC5/LConn3 -- Switches ABC6/LConn3
  Switches ABC7/LConn1 -- Switches ABC0/LConn1 -- A/RConn1 -- Switches ABC1/LConn1 -- Switches ABC2/LConn1 -- Switches ABC3/LConn1 -- Switches ABC4/LConn1 -- Switches ABC5/LConn1 -- Switches ABC6/LConn1

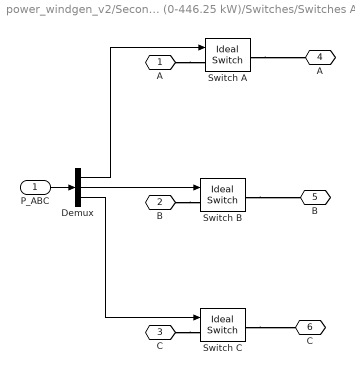
== system power_windgen_v2/Secondary Load (0-446.25 kW)/Switches/Switches ABC0 ==
  P_ABC : Inport
  Demux : Demux  Outputs=3
      settings: DisplayOption=none
  Switch A : spsIdealSwitchLib/Ideal Switch  Ron=Ron_switch  Lon=0  IC=Status(1)  Rs=Rs_snubber  Cs=Cs_snubber  Measurements=off
      settings: AttributesFormatString=\n
  Switch B : spsIdealSwitchLib/Ideal Switch  Ron=Ron_switch  Lon=0  IC=Status(1)  Rs=Rs_snubber  Cs=Cs_snubber  Measurements=off
      settings: AttributesFormatString=\n
  Switch C : spsIdealSwitchLib/Ideal Switch  Ron=Ron_switch  Lon=0  IC=Status(1)  Rs=Rs_snubber  Cs=Cs_snubber  Measurements=off
      settings: AttributesFormatString=\n
  A : PMIOPort  Side=Left
  B : PMIOPort  Port=2  Side=Left
  C : PMIOPort  Port=3  Side=Left
  "A " : PMIOPort  Port=4  Side=Right
  "B " : PMIOPort  Port=5  Side=Right
  "C " : PMIOPort  Port=6  Side=Right
  wires:
  P_ABC/1 -> Demux/1
  Demux/3 -> Switch C/1
  Demux/2 -> Switch B/1
  Demux/1 -> Switch A/1
  connections:
  Switch C/RConn1 -- "C "/RConn1
  Switch B/RConn1 -- "B "/RConn1
  Switch A/RConn1 -- "A "/RConn1
  C/RConn1 -- Switch C/LConn1
  B/RConn1 -- Switch B/LConn1
  A/RConn1 -- Switch A/LConn1

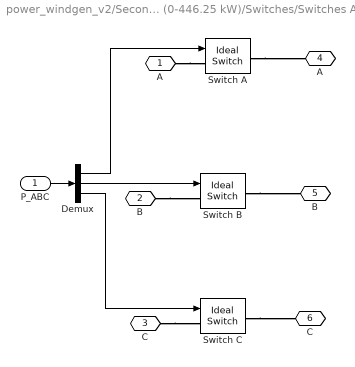
== system power_windgen_v2/Secondary Load (0-446.25 kW)/Switches/Switches ABC1 ==
  P_ABC : Inport
  Demux : Demux  Outputs=3
      settings: DisplayOption=none
  Switch A : spsIdealSwitchLib/Ideal Switch  Ron=Ron_switch  Lon=0  IC=Status(2)  Rs=Rs_snubber  Cs=Cs_snubber  Measurements=off
      settings: AttributesFormatString=\n
  Switch B : spsIdealSwitchLib/Ideal Switch  Ron=Ron_switch  Lon=0  IC=Status(2)  Rs=Rs_snubber  Cs=Cs_snubber  Measurements=off
      settings: AttributesFormatString=\n
  Switch C : spsIdealSwitchLib/Ideal Switch  Ron=Ron_switch  Lon=0  IC=Status(2)  Rs=Rs_snubber  Cs=Cs_snubber  Measurements=off
      settings: AttributesFormatString=\n
  A : PMIOPort  Side=Left
  B : PMIOPort  Port=2  Side=Left
  C : PMIOPort  Port=3  Side=Left
  "A " : PMIOPort  Port=4  Side=Right
  "B " : PMIOPort  Port=5  Side=Right
  "C " : PMIOPort  Port=6  Side=Right
  wires:
  Demux/1 -> Switch A/1
  Demux/2 -> Switch B/1
  Demux/3 -> Switch C/1
  P_ABC/1 -> Demux/1
  connections:
  A/RConn1 -- Switch A/LConn1
  B/RConn1 -- Switch B/LConn1
  Switch A/RConn1 -- "A "/RConn1
  Switch B/RConn1 -- "B "/RConn1
  Switch C/RConn1 -- "C "/RConn1
  C/RConn1 -- Switch C/LConn1

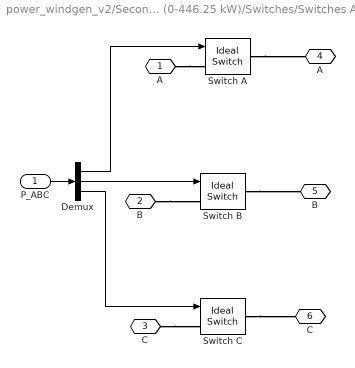
== system power_windgen_v2/Secondary Load (0-446.25 kW)/Switches/Switches ABC2 ==
  P_ABC : Inport
  Demux : Demux  Outputs=3
      settings: DisplayOption=none
  Switch A : spsIdealSwitchLib/Ideal Switch  Ron=Ron_switch  Lon=0  IC=Status(3)  Rs=Rs_snubber  Cs=Cs_snubber  Measurements=off
      settings: AttributesFormatString=\n
  Switch B : spsIdealSwitchLib/Ideal Switch  Ron=Ron_switch  Lon=0  IC=Status(3)  Rs=Rs_snubber  Cs=Cs_snubber  Measurements=off
      settings: AttributesFormatString=\n
  Switch C : spsIdealSwitchLib/Ideal Switch  Ron=Ron_switch  Lon=0  IC=Status(3)  Rs=Rs_snubber  Cs=Cs_snubber  Measurements=off
      settings: AttributesFormatString=\n
  A : PMIOPort  Side=Left
  B : PMIOPort  Port=2  Side=Left
  C : PMIOPort  Port=3  Side=Left
  "A " : PMIOPort  Port=4  Side=Right
  "B " : PMIOPort  Port=5  Side=Right
  "C " : PMIOPort  Port=6  Side=Right
  wires:
  P_ABC/1 -> Demux/1
  Demux/3 -> Switch C/1
  Demux/2 -> Switch B/1
  Demux/1 -> Switch A/1
  connections:
  Switch C/RConn1 -- "C "/RConn1
  Switch B/RConn1 -- "B "/RConn1
  Switch A/RConn1 -- "A "/RConn1
  A/RConn1 -- Switch A/LConn1
  B/RConn1 -- Switch B/LConn1
  C/RConn1 -- Switch C/LConn1

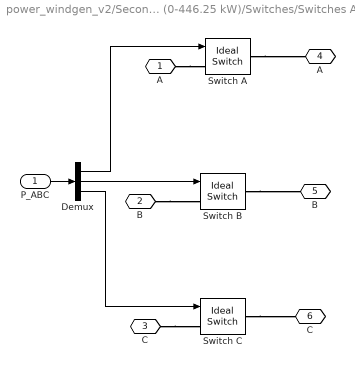
== system power_windgen_v2/Secondary Load (0-446.25 kW)/Switches/Switches ABC3 ==
  P_ABC : Inport
  Demux : Demux  Outputs=3
      settings: DisplayOption=none
  Switch A : spsIdealSwitchLib/Ideal Switch  Ron=Ron_switch  Lon=0  IC=Status(4)  Rs=Rs_snubber  Cs=Cs_snubber  Measurements=off
      settings: AttributesFormatString=\n
  Switch B : spsIdealSwitchLib/Ideal Switch  Ron=Ron_switch  Lon=0  IC=Status(4)  Rs=Rs_snubber  Cs=Cs_snubber  Measurements=off
      settings: AttributesFormatString=\n
  Switch C : spsIdealSwitchLib/Ideal Switch  Ron=Ron_switch  Lon=0  IC=Status(4)  Rs=Rs_snubber  Cs=Cs_snubber  Measurements=off
      settings: AttributesFormatString=\n
  A : PMIOPort  Side=Left
  B : PMIOPort  Port=2  Side=Left
  C : PMIOPort  Port=3  Side=Left
  "A " : PMIOPort  Port=4  Side=Right
  "B " : PMIOPort  Port=5  Side=Right
  "C " : PMIOPort  Port=6  Side=Right
  wires:
  Demux/1 -> Switch A/1
  Demux/2 -> Switch B/1
  Demux/3 -> Switch C/1
  P_ABC/1 -> Demux/1
  connections:
  C/RConn1 -- Switch C/LConn1
  B/RConn1 -- Switch B/LConn1
  A/RConn1 -- Switch A/LConn1
  Switch A/RConn1 -- "A "/RConn1
  Switch B/RConn1 -- "B "/RConn1
  Switch C/RConn1 -- "C "/RConn1

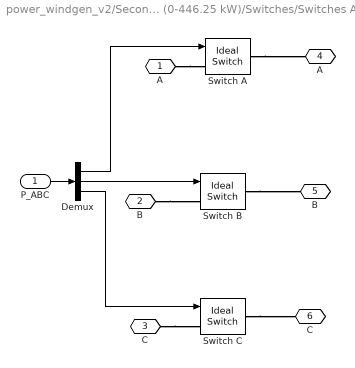
== system power_windgen_v2/Secondary Load (0-446.25 kW)/Switches/Switches ABC4 ==
  P_ABC : Inport
  Demux : Demux  Outputs=3
      settings: DisplayOption=none
  Switch A : spsIdealSwitchLib/Ideal Switch  Ron=Ron_switch  Lon=0  IC=Status(5)  Rs=Rs_snubber  Cs=Cs_snubber  Measurements=off
      settings: AttributesFormatString=\n
  Switch B : spsIdealSwitchLib/Ideal Switch  Ron=Ron_switch  Lon=0  IC=Status(5)  Rs=Rs_snubber  Cs=Cs_snubber  Measurements=off
      settings: AttributesFormatString=\n
  Switch C : spsIdealSwitchLib/Ideal Switch  Ron=Ron_switch  Lon=0  IC=Status(5)  Rs=Rs_snubber  Cs=Cs_snubber  Measurements=off
      settings: AttributesFormatString=\n
  A : PMIOPort  Side=Left
  B : PMIOPort  Port=2  Side=Left
  C : PMIOPort  Port=3  Side=Left
  "A " : PMIOPort  Port=4  Side=Right
  "B " : PMIOPort  Port=5  Side=Right
  "C " : PMIOPort  Port=6  Side=Right
  wires:
  P_ABC/1 -> Demux/1
  Demux/3 -> Switch C/1
  Demux/2 -> Switch B/1
  Demux/1 -> Switch A/1
  connections:
  Switch C/RConn1 -- "C "/RConn1
  Switch B/RConn1 -- "B "/RConn1
  Switch A/RConn1 -- "A "/RConn1
  A/RConn1 -- Switch A/LConn1
  B/RConn1 -- Switch B/LConn1
  C/RConn1 -- Switch C/LConn1

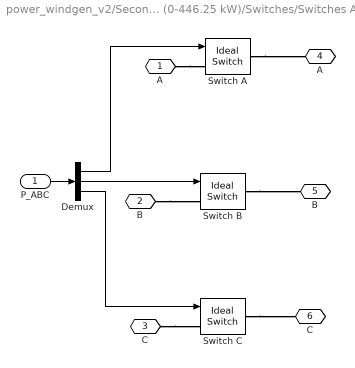
== system power_windgen_v2/Secondary Load (0-446.25 kW)/Switches/Switches ABC5 ==
  P_ABC : Inport
  Demux : Demux  Outputs=3
      settings: DisplayOption=none
  Switch A : spsIdealSwitchLib/Ideal Switch  Ron=Ron_switch  Lon=0  IC=Status(6)  Rs=Rs_snubber  Cs=Cs_snubber  Measurements=off
      settings: AttributesFormatString=\n
  Switch B : spsIdealSwitchLib/Ideal Switch  Ron=Ron_switch  Lon=0  IC=Status(6)  Rs=Rs_snubber  Cs=Cs_snubber  Measurements=off
      settings: AttributesFormatString=\n
  Switch C : spsIdealSwitchLib/Ideal Switch  Ron=Ron_switch  Lon=0  IC=Status(6)  Rs=Rs_snubber  Cs=Cs_snubber  Measurements=off
      settings: AttributesFormatString=\n
  A : PMIOPort  Side=Left
  B : PMIOPort  Port=2  Side=Left
  C : PMIOPort  Port=3  Side=Left
  "A " : PMIOPort  Port=4  Side=Right
  "B " : PMIOPort  Port=5  Side=Right
  "C " : PMIOPort  Port=6  Side=Right
  wires:
  Demux/1 -> Switch A/1
  Demux/2 -> Switch B/1
  Demux/3 -> Switch C/1
  P_ABC/1 -> Demux/1
  connections:
  C/RConn1 -- Switch C/LConn1
  B/RConn1 -- Switch B/LConn1
  A/RConn1 -- Switch A/LConn1
  Switch A/RConn1 -- "A "/RConn1
  Switch B/RConn1 -- "B "/RConn1
  Switch C/RConn1 -- "C "/RConn1

== system power_windgen_v2/Secondary Load (0-446.25 kW)/Switches/Switches ABC6 ==
  P_ABC : Inport
  Demux : Demux  Outputs=3
      settings: DisplayOption=none
  Switch A : spsIdealSwitchLib/Ideal Switch  Ron=Ron_switch  Lon=0  IC=Status(7)  Rs=Rs_snubber  Cs=Cs_snubber  Measurements=off
      settings: AttributesFormatString=\n
  Switch B : spsIdealSwitchLib/Ideal Switch  Ron=Ron_switch  Lon=0  IC=Status(7)  Rs=Rs_snubber  Cs=Cs_snubber  Measurements=off
      settings: AttributesFormatString=\n
  Switch C : spsIdealSwitchLib/Ideal Switch  Ron=Ron_switch  Lon=0  IC=Status(7)  Rs=Rs_snubber  Cs=Cs_snubber  Measurements=off
      settings: AttributesFormatString=\n
  A : PMIOPort  Side=Left
  B : PMIOPort  Port=2  Side=Left
  C : PMIOPort  Port=3  Side=Left
  "A " : PMIOPort  Port=4  Side=Right
  "B " : PMIOPort  Port=5  Side=Right
  "C " : PMIOPort  Port=6  Side=Right
  wires:
  P_ABC/1 -> Demux/1
  Demux/3 -> Switch C/1
  Demux/2 -> Switch B/1
  Demux/1 -> Switch A/1
  connections:
  Switch C/RConn1 -- "C "/RConn1
  Switch B/RConn1 -- "B "/RConn1
  Switch A/RConn1 -- "A "/RConn1
  A/RConn1 -- Switch A/LConn1
  B/RConn1 -- Switch B/LConn1
  C/RConn1 -- Switch C/LConn1

== system power_windgen_v2/Secondary Load (0-446.25 kW)/Switches/Switches ABC7 ==
  P_ABC : Inport
  Demux : Demux  Outputs=3
      settings: DisplayOption=none
  Switch A : spsIdealSwitchLib/Ideal Switch  Ron=Ron_switch  Lon=0  IC=Status(8)  Rs=Rs_snubber  Cs=Cs_snubber  Measurements=off
      settings: AttributesFormatString=\n
  Switch B : spsIdealSwitchLib/Ideal Switch  Ron=Ron_switch  Lon=0  IC=Status(8)  Rs=Rs_snubber  Cs=Cs_snubber  Measurements=off
      settings: AttributesFormatString=\n
  Switch C : spsIdealSwitchLib/Ideal Switch  Ron=Ron_switch  Lon=0  IC=Status(8)  Rs=Rs_snubber  Cs=Cs_snubber  Measurements=off
      settings: AttributesFormatString=\n
  A : PMIOPort  Side=Left
  B : PMIOPort  Port=2  Side=Left
  C : PMIOPort  Port=3  Side=Left
  "A " : PMIOPort  Port=4  Side=Right
  "B " : PMIOPort  Port=5  Side=Right
  "C " : PMIOPort  Port=6  Side=Right
  wires:
  Demux/1 -> Switch A/1
  Demux/2 -> Switch B/1
  Demux/3 -> Switch C/1
  P_ABC/1 -> Demux/1
  connections:
  C/RConn1 -- Switch C/LConn1
  B/RConn1 -- Switch B/LConn1
  A/RConn1 -- Switch A/LConn1
  Switch A/RConn1 -- "A "/RConn1
  Switch B/RConn1 -- "B "/RConn1
  Switch C/RConn1 -- "C "/RConn1
